simulink model "IP_LinearSys_LQG"  (R2015a)
settings: Solver=ode5  StartTime=0.0  StopTime=10  FixedStep=0.01  RelTol=1e-3
undefined symbols (not defined in the file): A, B, C, Continuous, D, Time, Ts
libraries: simulink x2, ctrlSharedLib x1
settings Model: Creator=Fares  LastModifiedBy=Fares

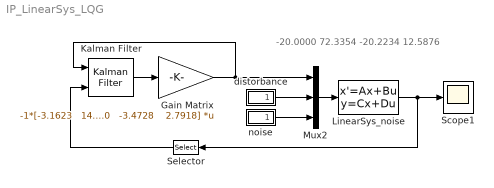
== system IP_LinearSys_LQG ==
  note: -20.0000 72.3354 -20.2234 12.5876
  Gain Matrix : Gain  Gain="-1*[-3.1623   14.6880   -3.4728    2.7918]"  Multiplication=Matrix(K*u) (u vector)
  Kalman Filter : ctrlSharedLib/Kalman Filter  TimeDomain=Continuous-Time  UseCurrentEstimator=on  ModelSource=Individual A, B, C, D matrices  ModelSourceVariable=ss(A,B,C,D,Ts)  A=A  B=B  C=C  D=D  NumberOfStates=1  NumberOfInputs=1  NumberOfOutputs=1  InitialEstimateSource=Dialog  X0=[0; 0; 0; 0]  P0=10  UseK=off  UseGH=off  NumberOfProcessNoiseInputs=1  G=1  TimeInvariantG=on  H=0  TimeInvariantH=on  Q=diag([0 0 0.1 0.1])  TimeInvariantQ=on  R=1e-04  TimeInvariantR=on  N=0  TimeInvariantN=on  AddInputPort=on  AddEnablePort=off  ExternalReset=none  OutputEstimatedY=off  OutputP=off  Ts=-1
  LinearSys_noise : StateSpace  A=A  B=BF  C=C  D=DF  X0=[0; 0; 0; 0]  mask(SS MASK){}
      mask init:
      | mc = 1.12;
      | mpw = 0.095;
      | mps = 0.025;
      | l = 0.033245968;
      | fc = 2.53165; % FS = 2.53165; FC = 2.28133
      | fp = 0.000107443;
      | J = 0.013935418;
      | g = 9.81;
      | vf = 9.4/2.5; %Voltage to Motor Force ratio
      | mp = mpw + mps;
      | a = l^2 + J/(mc + mp);
      | mu = (mc + mp)*l;
      | 
      | % theta 0 in upward position
      | % theta pi in downward position
      | s = -1; % 1 when upward  -1 when downward
      | 
      | A = [0          0              1               0;
      |      0          0              0               1;
      |      0      (l*mu*g)/J    -(a*fc)/J    -(l*fp)/J;
      |      0      s*(mu*g)/J    -s*(l*fc)/J    -(fp)/J];
      |  
      | B = [         0;
      |               0;
      |        (vf*a)/J;
      |       (s*vf*l)/J];
      |   
      | C = [1 0 0 0;
      |      0 1 0 0;
      |      0 0 1 0;
      |      0 0 0 1];
      |  
      | D = [0;
      |      0;
      |      0;
      |      0];
      |  
      | G = eye(4);
      | H = [1;
      |      0;
      |      0;
      |      0];
      |  
      | BF = [B G zeros(4,1)];
      | DF = [D zeros(4,4) H];
  Mux2 : Mux  Inputs=3
  Scope1 : Scope
      settings: ShowLegends=on  YMin=-0.19291  YMax=0.328423  SaveName=linSysNoise
  Selector : Selector  InputPortWidth=4  Indices=[1]
  distorbance : Subsystem
  noise : Subsystem
  wires:
  Kalman Filter/1 -> Gain Matrix/1
  LinearSys_noise/1 -> Selector/1, Scope1/1
  Selector/1 -> Kalman Filter/2
  Gain Matrix/1 -> Mux2/1, Kalman Filter/1
  distorbance/1(Out1) -> Mux2/2
  noise/1(Out1) -> Mux2/3
  Mux2/1 -> LinearSys_noise/1

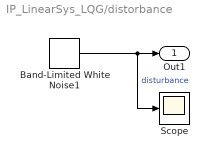
== system IP_LinearSys_LQG/distorbance ==
  Band-Limited White Noise1 : simulink/Sources/Band-Limited White Noise  Cov=[0 0 0.1*0.01 0.1*0.01]  Ts=0.01  seed=[23341]
  Scope : Scope
      settings: SaveName=noise
  Out1 : Outport
  wires:
  Band-Limited White Noise1/1 -> Scope/1, Out1/1  "disturbance"

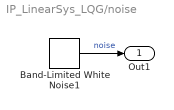
== system IP_LinearSys_LQG/noise ==
  Band-Limited White Noise1 : simulink/Sources/Band-Limited White Noise  Cov=[1e-4*0.01]  Ts=0.01  seed=[23341]
  Out1 : Outport
  wires:
  Band-Limited White Noise1/1 -> Out1/1  "noise"
